simulink model "FuncTransEjemMult"  (R2018a)
settings: Solver=VariableStepAuto  StartTime=0.0  StopTime=10.0  RelTol=1e-3
settings Model: Creator=adtenla  LastModifiedBy=adtenla

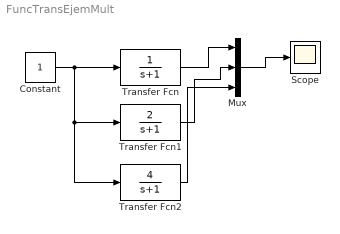
== system FuncTransEjemMult ==
  Constant : Constant
  Mux : Mux  Inputs=3
  Scope : Scope
  Transfer Fcn : TransferFcn  Denominator=[1 1]
  Transfer Fcn1 : TransferFcn  Numerator=[2]  Denominator=[1 1]
  Transfer Fcn2 : TransferFcn  Numerator=[4]  Denominator=[1 1]
  wires:
  Constant/1 -> Transfer Fcn/1, Transfer Fcn2/1, Transfer Fcn1/1
  Transfer Fcn/1 -> Mux/1
  Transfer Fcn1/1 -> Mux/2
  Transfer Fcn2/1 -> Mux/3
  Mux/1 -> Scope/1
